simulink model "power_controlvolt"  (Simulink 6.0)
settings: Solver=ode23tb  SolverMode=SingleTasking  StartTime=0.0  StopTime=0.1  MaxStep=1e-04  RelTol=1e-3  AbsTol=1e-6
libraries: powerlib x14
settings Model: Creator=patrice  LastModifiedBy=batserve  ExtModeTrigMode=oneshot  ExtModeArmWhenConnect=off  ExtModeAutoUpdateStatusClock=off
settings DataIOCC: LimitDataPoints=off  SignalLoggingName=sigsOut
settings OptimizationCC: BlockReduction=off  BooleanDataType=off
settings DebuggingCC: SolverPrmCheckMsg=none
settings HardwareCC: TargetUnknown=on
settings RTWCC: TemplateMakefile=grt_unix.tmf

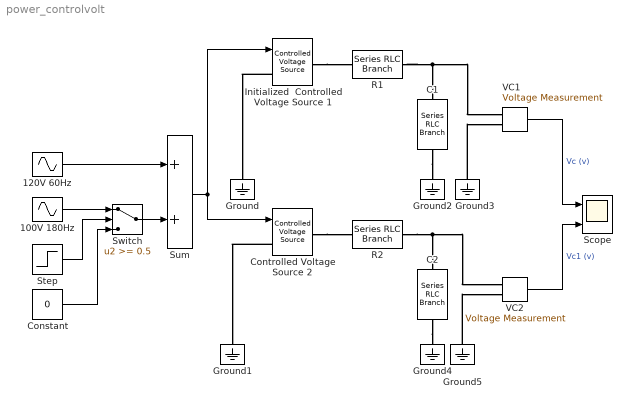
== system power_controlvolt ==
  100V 180Hz : Sin  Amplitude=100  Frequency=2*pi*180  SampleTime=0
  120V 60Hz : Sin  Amplitude=120  Frequency=2*pi*60  SampleTime=0
  C1 : powerlib/Elements/Series RLC Branch  Orientation=down  PhysicalDomain=powersysdomain  SubClassName=unknown  PortType=p1  LConnTagsString=__new0  RConnTagsString=__new0  Resistance=0  Inductance=0  Capacitance=500e-6  Measurements=None
  C2 : powerlib/Elements/Series RLC Branch  Orientation=down  PhysicalDomain=powersysdomain  SubClassName=unknown  PortType=p1  LConnTagsString=__new0  RConnTagsString=__new0  Resistance=0  Inductance=0  Capacitance=500e-6  Measurements=None
  Constant : Constant  Value=0
  Controlled Voltage Source 2 : powerlib/Electrical Sources/Controlled Voltage Source  Description=source block  Initialize=off  Amplitude=120  Phase=0  Frequency=60  Measurements=None
      settings: AttributesFormatString=\n
  Ground{,1..5} (6 alike) : powerlib/Elements/Ground  Orientation=down  PhysicalDomain=powersysdomain  SubClassName=unknown  PortType=p1  LConnTagsString=a
  Initialized  Controlled Voltage Source 1 : powerlib/Electrical Sources/Controlled Voltage Source  Description=source block  Initialize=on  Amplitude=120  Phase=0  Frequency=60  Measurements=None
      settings: AttributesFormatString=\n
  R1 : powerlib/Elements/Series RLC Branch  PhysicalDomain=powersysdomain  SubClassName=unknown  PortType=p1  LConnTagsString=__new0  RConnTagsString=__new0  Resistance=10  Inductance=0  Capacitance=inf  Measurements=None
  R2 : powerlib/Elements/Series RLC Branch  PhysicalDomain=powersysdomain  SubClassName=unknown  PortType=p1  LConnTagsString=__new0  RConnTagsString=__new0  Resistance=10  Inductance=0  Capacitance=inf  Measurements=None
  Scope : Scope  NumInputPorts=2
      settings: TickLabels=on  TimeRange=0.1  YMin=-100~-100  YMax=100~100  DataFormat=Array
  Step : Step  Time=2/60  SampleTime=0
  Sum : Sum  SaturateOnIntegerOverflow=on  InputSameDT=on
  Switch : Switch  Threshold=0.5  SaturateOnIntegerOverflow=on  InputSameDT=on
  VC1 : powerlib/Measurements/Voltage Measurement  Tag=PoWeRsYsTeMmEaSuReMeNt  PhasorSimulation=off  OutputType=Magnitude  PSBequivalent=0
  VC2 : powerlib/Measurements/Voltage Measurement  Tag=PoWeRsYsTeMmEaSuReMeNt  PhasorSimulation=off  OutputType=Magnitude  PSBequivalent=0
  wires:
  120V 60Hz/1 -> Sum/1
  Switch/1 -> Sum/2
  Step/1 -> Switch/2
  100V 180Hz/1 -> Switch/1
  Constant/1 -> Switch/3
  VC1/1 -> Scope/1  "Vc (v)"
  VC2/1 -> Scope/2  "Vc1 (v)"
  Sum/1 -> Initialized  Controlled Voltage Source 1/1, Controlled Voltage Source 2/1
  connections:
  Initialized  Controlled Voltage Source 1/LConn1 -- Ground/LConn1
  Initialized  Controlled Voltage Source 1/RConn1 -- R1/LConn1
  R1/RConn1 -- C1/LConn1 -- VC1/LConn1
  C1/RConn1 -- Ground2/LConn1
  Controlled Voltage Source 2/LConn1 -- Ground1/LConn1
  Controlled Voltage Source 2/RConn1 -- R2/LConn1
  R2/RConn1 -- VC2/LConn1 -- C2/LConn1
  C2/RConn1 -- Ground4/LConn1
  Ground3/LConn1 -- VC1/LConn2
  Ground5/LConn1 -- VC2/LConn2
